simulink model "ecal_helloworld_snd"  (R2021a)
settings: Solver=FixedStepDiscrete  StartTime=0.0  StopTime=inf  RelTol=1e-3
undefined symbols (not defined in the file): base, std
libraries: eCAL_blks_lib x1
settings Model: EnablePacing=on  Creator=uidp3321  LastModifiedBy=promero
settings SolverCC: ConcurrentTasks=on  AlgebraicLoopSolver=TrustRegion  PositivePriorityOrder=on
settings DataIOCC: ReturnWorkspaceOutputs=off
settings OptimizationCC: BlockReduction=off  OptimizeBlockIOStorage=off
settings DebuggingCC: TasksWithSamePriorityMsg=none  SFMachineParentedDataDiag=warning  ArithmeticOperatorsInVariantConditions=warning
settings HardwareCC: ProdBitPerLong=64  ProdLongLongMode=on  ProdHWDeviceType=Intel->x86-64 (Linux 64)
settings SFSimCC: SimUseLocalCustomCode=off  CustomCodeUndefinedFunction=UseInterfaceOnly  SimTargetLang=C++
settings RTWCC: Description=Simulink Real-Time  SystemTargetFile=slrealtime.tlc  TemplateMakefile=slrealtime_default_tmf  RTWUseLocalCustomCode=off  Toolchain=Simulink Real-Time Toolchain  BuildConfiguration=Faster Runs  CodeExecutionProfiling=on  TargetLang=C++
settings SimulinkRealTimeTargetCC: UseGCCFastMath=on

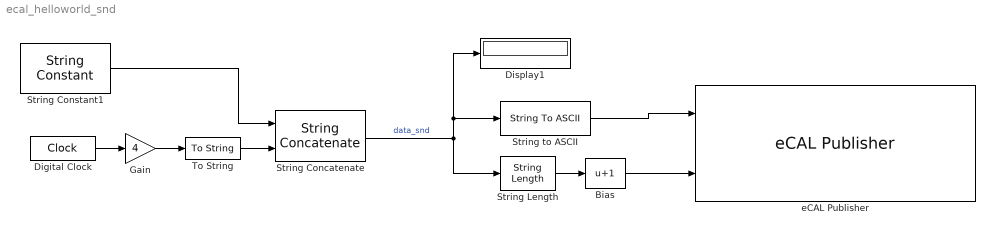
== system ecal_helloworld_snd ==
  Bias : Bias  Bias=1
  Digital Clock : DigitalClock  SampleTime=-1
  Display1 : Display
  Gain : Gain  Gain=4
  String Concatenate : StringConcatenate
  String Constant1 : StringConstant  String="\"Hello world: \""
  String Length : StringLength  OutDataTypeStr=uint32
  String to ASCII : StringToASCII  OutputVectorSize=50
  To String : ToString
  eCAL Publisher : eCAL_blks_lib/eCAL Publisher  param_topic_name=Hello  param_topic_type=base:std::string  param_signal_type=fixed  param_sample_time=0.25
      settings: SourceProductName=eCAL Blockset
  wires:
  Digital Clock/1 -> Gain/1
  Gain/1 -> To String/1
  String to ASCII/1 -> eCAL Publisher/1
  String Concatenate/1 -> Display1/1, String to ASCII/1, String Length/1  "data_snd"
  String Length/1 -> Bias/1
  Bias/1 -> eCAL Publisher/2
  String Constant1/1 -> String Concatenate/1
  To String/1 -> String Concatenate/2
